simulink model "GeneratedModelTestMyInput"  (R2014b)
settings: Solver=ode3  StartTime=0.0  StopTime=4.65  FixedStep=1/140  RelTol=1e-9
libraries: simulink x2
settings Model: Creator=levente.nagy960115  LastModifiedBy=NagyZe

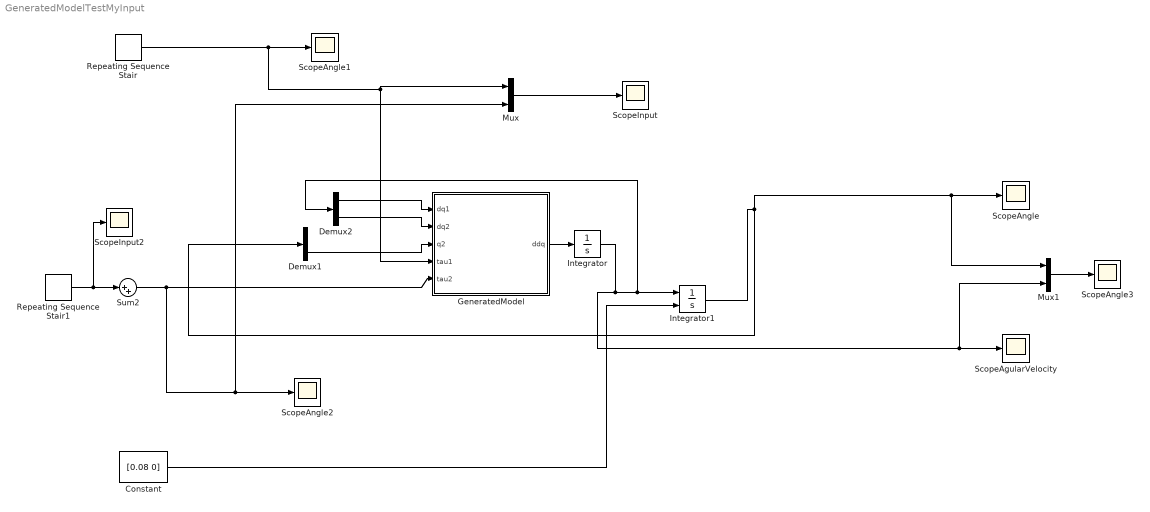
== system GeneratedModelTestMyInput ==
  Constant : Constant  Value=[0.08 0]
  Demux1 : Demux  Outputs=2
  Demux2 : Demux  Outputs=2
  GeneratedModel : MATLAB Function  TreatAsAtomicUnit=on
  Integrator : Integrator  InitialCondition=[0 0]
  Integrator1 : Integrator  InitialConditionSource=external  InitialCondition=[0 pi-0.1 0.1]
  Mux : Mux  Inputs=2
  Mux1 : Mux  Inputs=2
  Repeating Sequence Stair : simulink/Sources/Repeating Sequence Stair  OutValues=Input1  tsamp=1/140  OutMin=[]  OutMax=[]  OutDataTypeStr=double  OutputDataTypeScalingMode=double  OutDataType=fixdt(0,8)  ConRadixGroup=Best Precision: Vector-wise  OutScaling=2^-12
  Repeating Sequence Stair1 : simulink/Sources/Repeating Sequence Stair  OutValues=Input2  tsamp=1/140  OutMin=[]  OutMax=[]  OutDataTypeStr=double  OutputDataTypeScalingMode=double  OutDataType=fixdt(0,8)  ConRadixGroup=Best Precision: Vector-wise  OutScaling=2^-12
  ScopeAgularVelocity : Scope
      settings: TimeRange=10  YMin=-40  YMax=30  SaveName=jointVelocity
  ScopeAngle{,1..3} (4 alike) : Scope
      ScopeAngle settings: TimeRange=10  YMin=0  SaveName=jointAngles
      ScopeAngle1 settings: TimeRange=10  YMin=0  SaveName=jointAngles1
      ScopeAngle2 settings: TimeRange=10  YMin=0  SaveName=jointAngles2
      ScopeAngle3 settings: TimeRange=10  YMin=0  SaveName=SimulationStates
  ScopeInput : Scope
      settings: TimeRange=10  YMin=0  SaveName=jointInput
  ScopeInput2 : Scope
      settings: TimeRange=10  YMin=0  SaveName=inputT2
  Sum2 : Sum  Inputs=|++
  wires:
  GeneratedModel/1(ddq) -> Integrator/1
  Integrator/1 -> Mux1/2, ScopeAgularVelocity/1, Demux2/1, Integrator1/1
  Integrator1/1 -> Demux1/1, Mux1/1, ScopeAngle/1
  Constant/1 -> Integrator1/2
  Demux2/1 -> GeneratedModel/1(dq1)
  Demux2/2 -> GeneratedModel/2(dq2)
  Demux1/2 -> GeneratedModel/3(q2)
  Sum2/1 -> Mux/2, ScopeAngle2/1, GeneratedModel/5(tau2)
  Mux/1 -> ScopeInput/1
  Mux1/1 -> ScopeAngle3/1
  Repeating Sequence Stair1/1 -> ScopeInput2/1, Sum2/1
  Repeating Sequence Stair/1 -> Mux/1, GeneratedModel/4(tau1), ScopeAngle1/1

== matlab function GeneratedModelTestMyInput/GeneratedModel ==
  data: dq1 input; ddq output; dq2 input; q2 input; tau1 input; tau2 input
function ddq = GeneratedModel(dq1,dq2,q2,tau1,tau2)
%#codegen

%    This function was generated by the Symbolic Math Toolbox version 6.1.
%    19-Oct-2016 14:27:05

t2 = cos(q2);
t3 = t2.*1.899099681086028e17;
t4 = t2.^2;
t5 = t4.*1.164543691243047e17;
t6 = t3+t5+1.05575770741716e17;
t7 = 1.0./t6;
t8 = q2.*2.0;
t9 = sin(t8);
t10 = sin(q2);
ddq = [-dq1.*(t7.*6.935975771714791e18-dq2.*t7.*(t9.*1.164543691243047e17+t10.*1.899099681086028e17))+t7.*tau1.*7.378697629483821e19;dq2.*(-6.619898658808531)+tau2.*2.364249521003047e2-dq1.^2.*(t9.*1.86568958538629e-1+t10.*3.042505423588401e-1)];
